simulink model "sysgenTripleBuffer"  (Simulink 7.7)
settings: Solver=ode3  SolverMode=SingleTasking  StartTime=0.0  StopTime=inf  FixedStep=1  RelTol=1e-3
PreLoadFcn:
  | sysgenTripleBuffer_PreloadFcn
undefined symbols (not defined in the file or in its folder): c_hsync, c_image_cols, c_image_rows, c_vsync, c_word_size, gray, pixel_period, videoFrame
libraries: xbsIndex_r4 x101, simulink x4, dspsigattribs x3, dspbuff3 x3, dspmtrx3 x3, xbsCopyrightNotice_r4 x1, vipsnks x1, vipsrcs x1
(part 1 of 2)
settings Model: Creator=arvinds  LastModifiedBy=wayneh
settings OptimizationCC: InlineParams=on
settings ModelReferenceCC: ModelReferenceNumInstancesAllowed=Single
settings SFSimCC: SimParseCustomCode=off

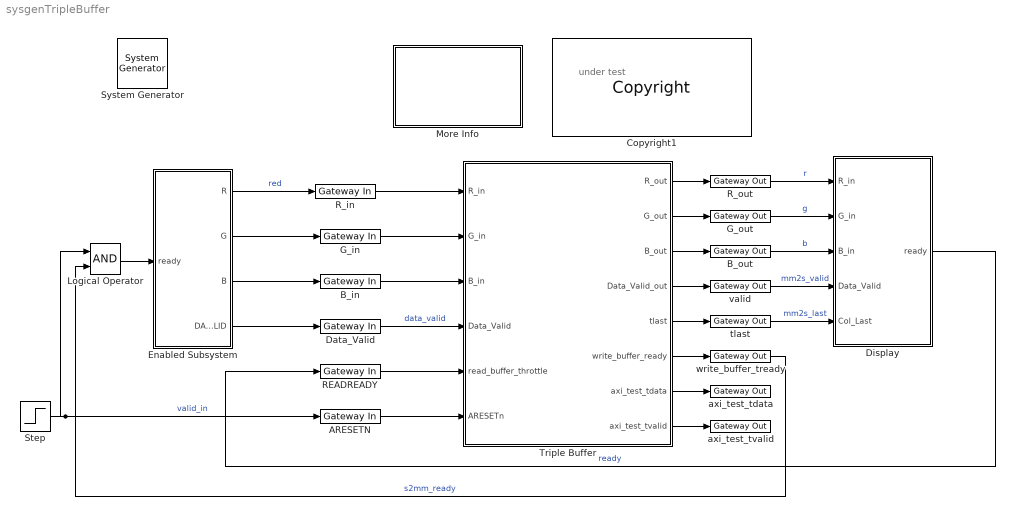
== system sysgenTripleBuffer ==
  note: under test
  " System Generator" : xbsIndex_r4/ System Generator  Tag=genX  SystemSampleTime=-1  xilinxfamily=virtex6  part=xc6vlx240t  speed=-1  package=ff1156  synthesis_tool=XST  clock_wrapper=Clock Enables  directory=./netlist_ml605_v5  proj_type=Project Navigator  Synth_file=XST Defaults  Impl_file=ISE Defaults  testbench=off  simulink_period=1  sysclk_period=20  dcm_input_clock_period=10  incr_netlist=off  trim_vbits=Everywhere in SubSystem  dbl_ovrd=According to Block Masks  core_generation=According to Block Masks  run_coregen=off  deprecated_control=off  eval_field=0  block_type=sysgen
      settings: block_version=12.3
  ARESETN : xbsIndex_r4/Gateway In  gui_display_data_type=Fixed-point  arith_type=Boolean  n_bits=8  bin_pt=0  preci_type=Single  exp_width=8  frac_width=24  quantization="Round  (unbiased: +/- Inf)"  overflow=Saturate  period=pixel_period  dbl_ovrd=off  timing_constraint=None  locs_specified=off  LOCs={}  inherit_from_input=off  UseAsADC=off  ADCChannel='1'  hdl_port=on  block_type=gatewayin
      settings: infoedit="Gateway in block.  Converts inputs of type Simulink integer, double and fixed point to  Xilinx fixed point type.<br><br>Hardware notes:  In hardware these blocks become top level input ports."  block_version=12.3
  B_in : xbsIndex_r4/Gateway In  gui_display_data_type=Fixed-point  arith_type=Unsigned  n_bits=8  bin_pt=0  preci_type=Single  exp_width=8  frac_width=24  quantization="Round  (unbiased: +/- Inf)"  overflow=Saturate  period=pixel_period  dbl_ovrd=off  timing_constraint=None  locs_specified=off  LOCs={}  inherit_from_input=off  UseAsADC=off  ADCChannel='1'  hdl_port=on  block_type=gatewayin
      settings: infoedit="Gateway in block.  Converts inputs of type Simulink integer, double and fixed point to  Xilinx fixed point type.<br><br>Hardware notes:  In hardware these blocks become top level input ports."  block_version=12.3
  B_out : xbsIndex_r4/Gateway Out  inherit_from_input=off  hdl_port=on  timing_constraint=None  locs_specified=off  LOCs={}  UseAsDAC=off  DACChannel='1'  block_type=gatewayout
      settings: infoedit="Gateway out block.  Converts Xilinx fixed point inputs into ouputs of type Simulink integer, double, or fixed point.<br><br>Hardware notes:  In hardware these blocks become top level output ports or are discarded, depending on how they are configured."  block_version=12.3
  Copyright1 : xbsCopyrightNotice_r4/Copyright  copyrighttext="Copyright (c) 2011  by  Xilinx, Inc. All rights reserved.<br><br>This file contains proprietary, confidential information of Xilinx, Inc., is distributed under license from Xilinx, Inc., and may be used, copied and/or disclosed only pursuant to the terms of a valid license agreement with Xilinx, Inc. Xilinx hereby grants you a license to use this file solely for design, simulation, implementation and creation of design files limited to Xilinx devices or technologies. Use with non-Xilinx devices or technologies is expressly prohibited and immediately terminates your license unless covered by a separate agreement.<br><br>Xilinx is providing this design, code, or information \"as-is\" solely for use in developing programs and solutions for Xilinx devices, with no obligation on the part of Xilinx to provide support. By providing this design, code, or information as one possible implementation of this feature, application or standard, Xilinx is making no representation that this implementation is free from any claims of infringement. You are responsible for obtaining any rights you may require for your implementation. Xilinx expressly disclaims any warranty whatsoever with respect to the adequacy of the implementation, including but not limited to any warranties or representations that this implementation is free from claims of infringement, implied warranties of merchantability or fitness for a particular purpose.<br><br>Xilinx products are not intended for use in life support appliances, devices, or systems. Use in such applications is expressly prohibited.<br><br>Any modifications that are made to the Source Code are done at the user's sole risk and will be unsupported.<br><br>This copyright and support notice must be retained as part of this text at all times. (c) Copyright 1995-2011 Xilinx, Inc. All rights reserved."  block_type=copyright
      settings: block_version=10.1.00
  Data_Valid : xbsIndex_r4/Gateway In  gui_display_data_type=Fixed-point  arith_type=Boolean  n_bits=8  bin_pt=0  preci_type=Single  exp_width=8  frac_width=24  quantization="Round  (unbiased: +/- Inf)"  overflow=Saturate  period=pixel_period  dbl_ovrd=off  timing_constraint=None  locs_specified=off  LOCs={}  inherit_from_input=off  UseAsADC=off  ADCChannel='1'  hdl_port=on  block_type=gatewayin
      settings: infoedit="Gateway in block.  Converts inputs of type Simulink integer, double and fixed point to  Xilinx fixed point type.<br><br>Hardware notes:  In hardware these blocks become top level input ports."  block_version=12.3
  Display : Subsystem  mask{im_rows=c_image_rows, im_cols=c_image_cols}
      mask prompts: im_rows "Image Rows"; im_cols "Image Cols"
  Enabled Subsystem : Subsystem  mask{image_cols=c_image_cols, image_rows=c_image_rows, vsync=c_vsync, hsync=c_hsync, videoFrame=videoFrame}
      mask prompts: image_cols "Image Cols"; image_rows "Image Rows"; vsync "VSYNC Size(rows)"; hsync "HSync Size (cols)"; videoFrame "Video Source"
  G_in : xbsIndex_r4/Gateway In  gui_display_data_type=Fixed-point  arith_type=Unsigned  n_bits=8  bin_pt=0  preci_type=Single  exp_width=8  frac_width=24  quantization="Round  (unbiased: +/- Inf)"  overflow=Saturate  period=pixel_period  dbl_ovrd=off  timing_constraint=None  locs_specified=off  LOCs={}  inherit_from_input=off  UseAsADC=off  ADCChannel='1'  hdl_port=on  block_type=gatewayin
      settings: infoedit="Gateway in block.  Converts inputs of type Simulink integer, double and fixed point to  Xilinx fixed point type.<br><br>Hardware notes:  In hardware these blocks become top level input ports."  block_version=12.3
  G_out : xbsIndex_r4/Gateway Out  inherit_from_input=off  hdl_port=on  timing_constraint=None  locs_specified=off  LOCs={}  UseAsDAC=off  DACChannel='1'  block_type=gatewayout
      settings: infoedit="Gateway out block.  Converts Xilinx fixed point inputs into ouputs of type Simulink integer, double, or fixed point.<br><br>Hardware notes:  In hardware these blocks become top level output ports or are discarded, depending on how they are configured."  block_version=12.3
  Logical Operator : Logic  AllPortsSameDT=off  OutDataTypeStr=boolean
  More Info : Subsystem
      mask Display: disp('Double click\n for\n more information.')
  READREADY : xbsIndex_r4/Gateway In  gui_display_data_type=Fixed-point  arith_type=Boolean  n_bits=8  bin_pt=0  preci_type=Single  exp_width=8  frac_width=24  quantization="Round  (unbiased: +/- Inf)"  overflow=Saturate  period=pixel_period  dbl_ovrd=off  timing_constraint=None  locs_specified=off  LOCs={}  inherit_from_input=off  UseAsADC=off  ADCChannel='1'  hdl_port=on  block_type=gatewayin
      settings: infoedit="Gateway in block.  Converts inputs of type Simulink integer, double and fixed point to  Xilinx fixed point type.<br><br>Hardware notes:  In hardware these blocks become top level input ports."  block_version=12.3
  R_in : xbsIndex_r4/Gateway In  gui_display_data_type=Fixed-point  arith_type=Unsigned  n_bits=8  bin_pt=0  preci_type=Single  exp_width=8  frac_width=24  quantization="Round  (unbiased: +/- Inf)"  overflow=Saturate  period=pixel_period  dbl_ovrd=off  timing_constraint=None  locs_specified=off  LOCs={}  inherit_from_input=off  UseAsADC=off  ADCChannel='1'  hdl_port=on  block_type=gatewayin
      settings: infoedit="Gateway in block.  Converts inputs of type Simulink integer, double and fixed point to  Xilinx fixed point type.<br><br>Hardware notes:  In hardware these blocks become top level input ports."  block_version=12.3
  R_out : xbsIndex_r4/Gateway Out  inherit_from_input=off  hdl_port=on  timing_constraint=None  locs_specified=off  LOCs={}  UseAsDAC=off  DACChannel='1'  block_type=gatewayout
      settings: infoedit="Gateway out block.  Converts Xilinx fixed point inputs into ouputs of type Simulink integer, double, or fixed point.<br><br>Hardware notes:  In hardware these blocks become top level output ports or are discarded, depending on how they are configured."  block_version=12.3
  Step : Step  Time=pixel_period*32  SampleTime=pixel_period
  Triple Buffer : Subsystem  mask{c_image_rows=c_image_rows, c_image_cols=c_image_cols, c_word_size=c_word_size}
      mask prompts: c_image_rows "Number of Rows"; c_image_cols "Number of Cols"; c_word_size "Pixel Size(In Bytes)"
  axi_test_tdata : xbsIndex_r4/Gateway Out  inherit_from_input=off  hdl_port=on  timing_constraint=None  locs_specified=off  LOCs={}  UseAsDAC=off  DACChannel='1'  block_type=gatewayout
      settings: infoedit="Gateway out block.  Converts Xilinx fixed point inputs into ouputs of type Simulink integer, double, or fixed point.<br><br>Hardware notes:  In hardware these blocks become top level output ports or are discarded, depending on how they are configured."  block_version=12.3
  axi_test_tvalid : xbsIndex_r4/Gateway Out  inherit_from_input=off  hdl_port=on  timing_constraint=None  locs_specified=off  LOCs={}  UseAsDAC=off  DACChannel='1'  block_type=gatewayout
      settings: infoedit="Gateway out block.  Converts Xilinx fixed point inputs into ouputs of type Simulink integer, double, or fixed point.<br><br>Hardware notes:  In hardware these blocks become top level output ports or are discarded, depending on how they are configured."  block_version=12.3
  tlast : xbsIndex_r4/Gateway Out  inherit_from_input=off  hdl_port=on  timing_constraint=None  locs_specified=off  LOCs={}  UseAsDAC=off  DACChannel='1'  block_type=gatewayout
      settings: infoedit="Gateway out block.  Converts Xilinx fixed point inputs into ouputs of type Simulink integer, double, or fixed point.<br><br>Hardware notes:  In hardware these blocks become top level output ports or are discarded, depending on how they are configured."  block_version=12.3
  valid : xbsIndex_r4/Gateway Out  inherit_from_input=off  hdl_port=on  timing_constraint=None  locs_specified=off  LOCs={}  UseAsDAC=off  DACChannel='1'  block_type=gatewayout
      settings: infoedit="Gateway out block.  Converts Xilinx fixed point inputs into ouputs of type Simulink integer, double, or fixed point.<br><br>Hardware notes:  In hardware these blocks become top level output ports or are discarded, depending on how they are configured."  block_version=12.3
  write_buffer_tready : xbsIndex_r4/Gateway Out  inherit_from_input=off  hdl_port=on  timing_constraint=None  locs_specified=off  LOCs={}  UseAsDAC=off  DACChannel='1'  block_type=gatewayout
      settings: infoedit="Gateway out block.  Converts Xilinx fixed point inputs into ouputs of type Simulink integer, double, or fixed point.<br><br>Hardware notes:  In hardware these blocks become top level output ports or are discarded, depending on how they are configured."  block_version=12.3
  wires:
  Step/1 -> Logical Operator/1, ARESETN/1  "valid_in"
  Enabled Subsystem/1(R) -> R_in/1  "red"
  Enabled Subsystem/2(G) -> G_in/1
  Enabled Subsystem/3(B) -> B_in/1
  R_out/1 -> Display/1(R_in)  "r"
  G_out/1 -> Display/2(G_in)  "g"
  B_out/1 -> Display/3(B_in)  "b"
  valid/1 -> Display/4(Data_Valid)  "mm2s_valid"
  tlast/1 -> Display/5(Col_Last)  "mm2s_last"
  write_buffer_tready/1 -> Logical Operator/2  "s2mm_ready"
  Enabled Subsystem/4(DATA_VALID) -> Data_Valid/1
  Logical Operator/1 -> Enabled Subsystem/1(ready)
  Display/1(ready) -> READREADY/1  "ready"
  R_in/1 -> Triple Buffer/1(R_in)
  G_in/1 -> Triple Buffer/2(G_in)
  B_in/1 -> Triple Buffer/3(B_in)
  Data_Valid/1 -> Triple Buffer/4(Data_Valid)  "data_valid"
  Triple Buffer/3(B_out) -> B_out/1
  Triple Buffer/4(Data_Valid_out) -> valid/1
  Triple Buffer/5(tlast) -> tlast/1
  Triple Buffer/6(write_buffer_ready) -> write_buffer_tready/1
  ARESETN/1 -> Triple Buffer/6(ARESETn)
  Triple Buffer/1(R_out) -> R_out/1
  Triple Buffer/2(G_out) -> G_out/1
  READREADY/1 -> Triple Buffer/5(read_buffer_throttle)
  Triple Buffer/7(axi_test_tdata) -> axi_test_tdata/1
  Triple Buffer/8(axi_test_tvalid) -> axi_test_tvalid/1

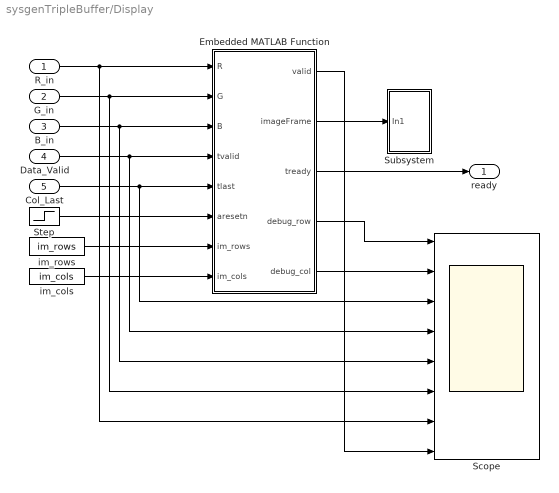
== system sysgenTripleBuffer/Display ==
  R_in : Inport
  G_in : Inport  Port=2
  B_in : Inport  Port=3
  Data_Valid : Inport  Port=4
  Col_Last : Inport  Port=5
  Embedded MATLAB Function : Stateflow chart  TreatAsAtomicUnit=on
  Scope : Scope  NumInputPorts=8
      settings: YMin=7.6~17.5~-1~0.95~-1~-1~-1~-1  YMax=8.4~35~1~1.05~1~1~1~1
  Step : Step  Time=pixel_period  SampleTime=pixel_period
  Subsystem : Subsystem
  im_cols : Constant  Value=im_cols
  im_rows : Constant  Value=im_rows
  ready : Outport
  wires:
  Step/1 -> Embedded MATLAB Function/6(aresetn)
  Embedded MATLAB Function/1(valid) -> Scope/8
  Embedded MATLAB Function/2(imageFrame) -> Subsystem/1(In1)
  R_in/1 -> Embedded MATLAB Function/1(R), Scope/7
  G_in/1 -> Embedded MATLAB Function/2(G), Scope/6
  B_in/1 -> Embedded MATLAB Function/3(B), Scope/5
  Col_Last/1 -> Embedded MATLAB Function/5(tlast), Scope/3
  Data_Valid/1 -> Embedded MATLAB Function/4(tvalid), Scope/4
  Embedded MATLAB Function/3(tready) -> ready/1
  im_rows/1 -> Embedded MATLAB Function/7(im_rows)
  im_cols/1 -> Embedded MATLAB Function/8(im_cols)
  Embedded MATLAB Function/4(debug_row) -> Scope/1
  Embedded MATLAB Function/5(debug_col) -> Scope/2

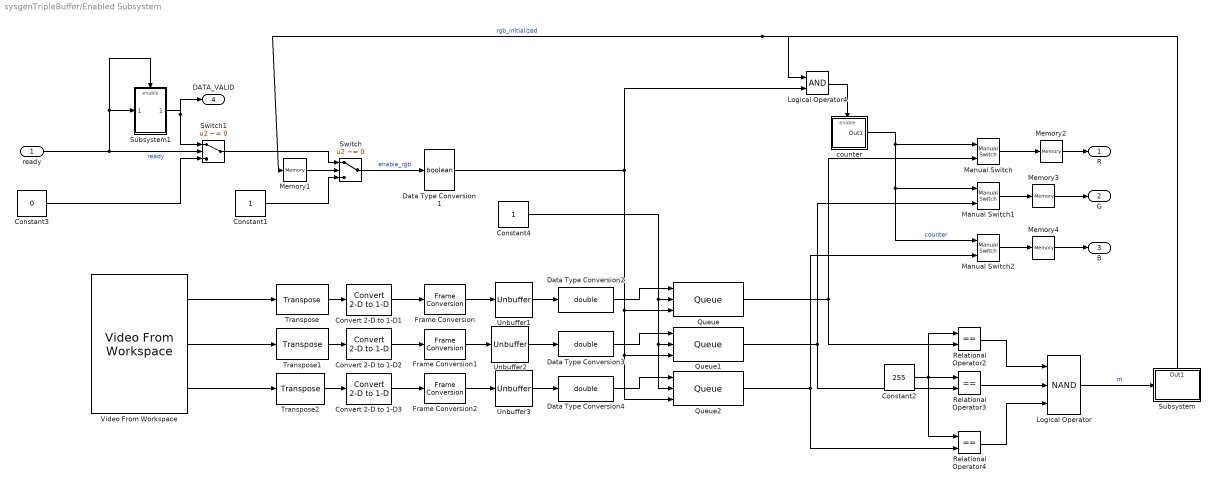
== system sysgenTripleBuffer/Enabled Subsystem ==
  ready : Inport
  Constant1 : Constant
  Constant2 : Constant  Value=255
  Constant3 : Constant  Value=0
  Constant4 : Constant  OutDataTypeStr=boolean
  Convert 2-D to 1-D1 : dspsigattribs/Convert 2-D to 1-D  SystemSampleTime=-1
  Convert 2-D to 1-D2 : dspsigattribs/Convert 2-D to 1-D  SystemSampleTime=-1
  Convert 2-D to 1-D3 : dspsigattribs/Convert 2-D to 1-D  SystemSampleTime=-1
  Data Type Conversion1 : DataTypeConversion  OutDataTypeStr=boolean
  Data Type Conversion2 : DataTypeConversion  OutDataTypeStr=double
  Data Type Conversion3 : DataTypeConversion  OutDataTypeStr=double
  Data Type Conversion4 : DataTypeConversion  OutDataTypeStr=double
  Frame Conversion : FrameConversion
  Frame Conversion1 : FrameConversion
  Frame Conversion2 : FrameConversion
  Logical Operator : Logic  Operator=NAND  Inputs=3  AllPortsSameDT=off  OutDataTypeStr=boolean
  Logical Operator4 : Logic  AllPortsSameDT=off  OutDataTypeStr=boolean
  Manual Switch : simulink/Signal Routing/Manual Switch  SystemSampleTime=-1  sw=0  action=0  varsize=off
  Manual Switch1 : simulink/Signal Routing/Manual Switch  SystemSampleTime=-1  sw=0  action=0  varsize=off
  Manual Switch2 : simulink/Signal Routing/Manual Switch  SystemSampleTime=-1  sw=0  action=0  varsize=off
  Memory{1..4} (4 alike) : Memory  InheritSampleTime=on  LinearizeMemory=on  LinearizeAsDelay=on
  Queue : dspbuff3/Queue  depth=image_cols*image_rows*10  trigger=Non-zero sample  overflow=Dynamic reallocation  pes=Warning  eso=off  fso=off  nso=off  clr=off  clrOutport=off  adf=on
  Queue1 : dspbuff3/Queue  depth=image_cols*image_rows*10  trigger=Non-zero sample  overflow=Dynamic reallocation  pes=Warning  eso=off  fso=off  nso=off  clr=off  clrOutport=off  adf=on
  Queue2 : dspbuff3/Queue  depth=image_cols*image_rows*10  trigger=Non-zero sample  overflow=Dynamic reallocation  pes=Warning  eso=off  fso=off  nso=off  clr=off  clrOutport=off  adf=on
  Relational Operator2 : RelationalOperator  Operator===  OutDataTypeStr=boolean
  Relational Operator3 : RelationalOperator  Operator===  OutDataTypeStr=boolean
  Relational Operator4 : RelationalOperator  Operator===  OutDataTypeStr=boolean
  Subsystem : Subsystem
  Subsystem1 : Subsystem
  Switch : Switch  Criteria=u2 ~= 0
  Switch1 : Switch  Criteria=u2 ~= 0
  Transpose : dspmtrx3/Transpose  SystemSampleTime=-1  Hermitian=off  overflowFlag=off
  Transpose1 : dspmtrx3/Transpose  SystemSampleTime=-1  Hermitian=off  overflowFlag=off
  Transpose2 : dspmtrx3/Transpose  SystemSampleTime=-1  Hermitian=off  overflowFlag=off
  Unbuffer1 : Unbuffer
  Unbuffer2 : Unbuffer
  Unbuffer3 : Unbuffer
  Video From Workspace : vipsrcs/Video From Workspace  signal=videoFrame  Ts=image_cols*image_rows  finalout=Obsolete  finaloutActive=Cyclic repetition  imagePorts=Separate color signals  OutPortLabels=R|G|B
  counter : Subsystem
  R : Outport
  G : Outport  Port=2
  B : Outport  Port=3
  DATA_VALID : Outport  Port=4  SampleTime=pixel_period
  wires:
  Relational Operator2/1 -> Logical Operator/1
  Relational Operator3/1 -> Logical Operator/2
  Relational Operator4/1 -> Logical Operator/3
  Subsystem/1(Out1) -> Logical Operator4/1, Memory1/1  "rgb_initialized"
  Constant1/1 -> Switch/3
  Switch/1 -> Data Type Conversion1/1  "enable_rgb"
  Manual Switch/1 -> Memory2/1
  Manual Switch1/1 -> Memory3/1
  Manual Switch2/1 -> Memory4/1
  counter/1(Out1) -> Manual Switch/1, Manual Switch1/1, Manual Switch2/1  "counter"
  Logical Operator4/1 -> counter/Enable
  Logical Operator/1 -> Subsystem/Enable  "m"
  Constant2/1 -> Relational Operator3/1, Relational Operator2/1, Relational Operator4/1
  Memory1/1 -> Switch/2
  ready/1 -> Subsystem1/1(In1), Subsystem1/Enable, Switch1/2  "ready"
  Subsystem1/1(Out1) -> Switch1/1, DATA_VALID/1
  Constant3/1 -> Switch1/3
  Switch1/1 -> Switch/1
  Convert 2-D to 1-D3/1 -> Frame Conversion2/1
  Transpose2/1 -> Convert 2-D to 1-D3/1
  Convert 2-D to 1-D2/1 -> Frame Conversion1/1
  Transpose1/1 -> Convert 2-D to 1-D2/1
  Convert 2-D to 1-D1/1 -> Frame Conversion/1
  Transpose/1 -> Convert 2-D to 1-D1/1
  Video From Workspace/1 -> Transpose/1
  Video From Workspace/2 -> Transpose1/1
  Video From Workspace/3 -> Transpose2/1
  Data Type Conversion1/1 -> Logical Operator4/2, Queue/3, Queue1/3, Queue2/3
  Data Type Conversion2/1 -> Queue/1
  Data Type Conversion3/1 -> Queue1/1
  Data Type Conversion4/1 -> Queue2/1
  Queue/1 -> Relational Operator2/2, Manual Switch/2
  Queue1/1 -> Relational Operator3/2, Manual Switch1/2
  Queue2/1 -> Relational Operator4/2, Manual Switch2/2
  Constant4/1 -> Queue/2, Queue1/2, Queue2/2
  Frame Conversion/1 -> Unbuffer1/1
  Frame Conversion1/1 -> Unbuffer2/1
  Frame Conversion2/1 -> Unbuffer3/1
  Unbuffer1/1 -> Data Type Conversion2/1
  Unbuffer2/1 -> Data Type Conversion3/1
  Unbuffer3/1 -> Data Type Conversion4/1
  Memory2/1 -> R/1
  Memory3/1 -> G/1
  Memory4/1 -> B/1

== system sysgenTripleBuffer/More Info ==
  note: Triple Buffer Demo
  note: This model implements a triple buffer controller that controls how frames are written to an external memory and read using a VDMA Interface 4.0 .
      | As the name suggests, triple buffer is a methodology used to synchronize data transfer between a writing device and reading device using
      | three buffers. The writing device does not write to the buffer that is being used by the reading device. Instead the writing device writes alternatively
      | to two buffers available to it. When the reading device has finished reading the buffer is swapped with the buffer that was last written to and the
      | process is continued. This methodology is generally used in graphics processing where the graphics processor is the writing device and
      | the display device is the reading device.
      |
      | The design can be netlisted using HDL Netlist in which case the VDMA Interface 4.0  block will be translated into top level gateways. Furthermore,
      | xlVDMACreateProject function can be used to create an ISE project to stitch SysGen design with VDMA Interface 3.0  & External Memory in XPS.
      | For more information please type the following in matlab console :
      | >>help xlVDMACreateProject
      |
      | Please refer to in case stateflow block compiler setup error.
      | http://www.mathworks.com/help/toolbox/stateflow/gs/bqnop_7-1.html

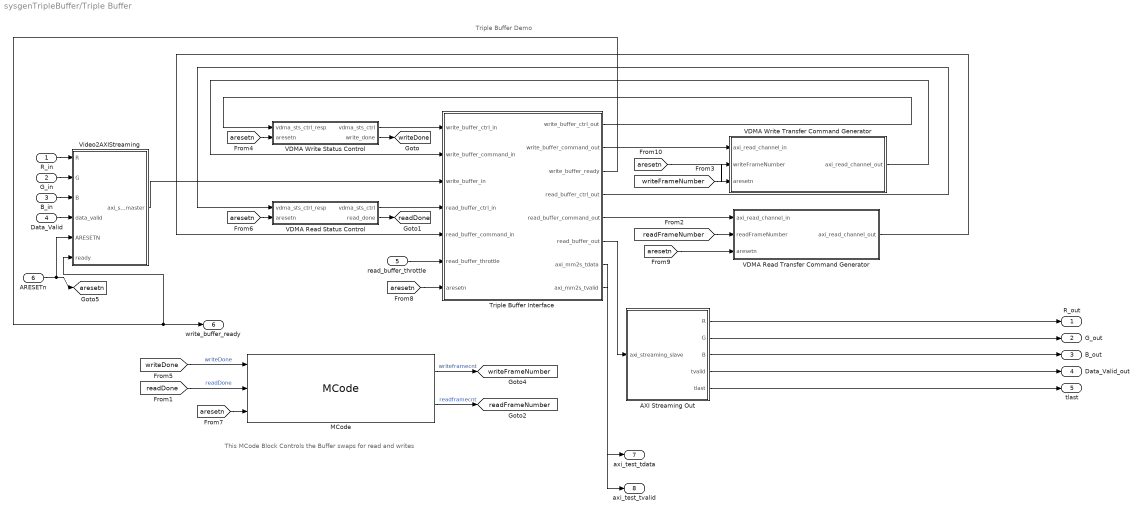
== system sysgenTripleBuffer/Triple Buffer ==
  note: This MCode Block Controls the Buffer swaps
      | for read and writes
  note: Triple Buffer Demo
  R_in : Inport
  G_in : Inport  Port=2
  B_in : Inport  Port=3
  Data_Valid : Inport  Port=4
  read_buffer_throttle : Inport  Port=5
  ARESETn : Inport  Port=6
  AXI Streaming Out : Subsystem
  MCode : xbsIndex_r4/MCode  mfname=xlTripleBufferAddressController  explicit_period=on  period=pixel_period  inputsTable={'boundInpExpr'=>['','',''],'inputs'=>['writeDone','readDone','aresetn']}  outputsTable={'outputs'=>['writeFrameNumber','readFrameNumber'],'suppressOut'=>['off','off']}  dbl_ovrd=off  enable_stdout=off  enable_debug=off  suppress_output=on  defparams={}  hide_port_list={}  block_type=mcode
      settings: block_version=12.3
  Triple Buffer Interface : Subsystem
  VDMA Read Status Control : Subsystem
  VDMA Read Transfer Command Generator : Subsystem
  VDMA Write Status Control : Subsystem
  VDMA Write Transfer Command Generator : Subsystem
  Video2AXIStreaming : Subsystem
  R_out : Outport
  G_out : Outport  Port=2
  B_out : Outport  Port=3
  Data_Valid_out : Outport  Port=4
  tlast : Outport  Port=5
  write_buffer_ready : Outport  Port=6
  axi_test_tdata : Outport  Port=7
  axi_test_tvalid : Outport  Port=8
  tag scope: aresetn=global, readDone=global, readFrameNumber=global, writeDone=global, writeFrameNumber=global
  wires:
  VDMA Write Status Control/1(vdma_sts_ctrl) -> Triple Buffer Interface/1(write_buffer_ctrl_in)
  Triple Buffer Interface/1(write_buffer_ctrl_out) -> VDMA Write Status Control/1(vdma_sts_ctrl_resp)
  VDMA Read Status Control/1(vdma_sts_ctrl) -> Triple Buffer Interface/4(read_buffer_ctrl_in)
  Triple Buffer Interface/4(read_buffer_ctrl_out) -> VDMA Read Status Control/1(vdma_sts_ctrl_resp)
  VDMA Write Status Control/2(write_done) -> [writeDone]
  VDMA Read Status Control/2(read_done) -> [readDone]
  [writeDone] -> MCode/1  "writeDone"
  [readDone] -> MCode/2  "readDone"
  Triple Buffer Interface/2(write_buffer_command_out) -> VDMA Write Transfer Command Generator/1(axi_read_channel_in)
  VDMA Write Transfer Command Generator/1(axi_read_channel_out) -> Triple Buffer Interface/2(write_buffer_command_in)
  Triple Buffer Interface/5(read_buffer_command_out) -> VDMA Read Transfer Command Generator/1(axi_read_channel_in)
  [readFrameNumber] -> VDMA Read Transfer Command Generator/2(readFrameNumber)
  [writeFrameNumber] -> VDMA Write Transfer Command Generator/2(writeFrameNumber)
  MCode/1 -> [writeFrameNumber]  "writeframecnt"
  [aresetn] -> VDMA Write Status Control/2(aresetn)
  ARESETn/1 -> Video2AXIStreaming/5(ARESETN), [aresetn]
  VDMA Read Transfer Command Generator/1(axi_read_channel_out) -> Triple Buffer Interface/5(read_buffer_command_in)
  [aresetn] -> MCode/3
  [aresetn] -> Triple Buffer Interface/7(aresetn)
  [aresetn] -> VDMA Write Transfer Command Generator/3(aresetn)
  [aresetn] -> VDMA Read Transfer Command Generator/3(aresetn)
  MCode/2 -> [readFrameNumber]  "readframecnt"
  [aresetn] -> VDMA Read Status Control/2(aresetn)
  Video2AXIStreaming/1(axi_streaming_master) -> Triple Buffer Interface/3(write_buffer_in)
  Triple Buffer Interface/6(read_buffer_out) -> AXI Streaming Out/1(axi_streaming_slave)
  AXI Streaming Out/1(R) -> R_out/1
  AXI Streaming Out/2(G) -> G_out/1
  AXI Streaming Out/3(B) -> B_out/1
  AXI Streaming Out/5(tlast) -> tlast/1
  AXI Streaming Out/4(tvalid) -> Data_Valid_out/1
  R_in/1 -> Video2AXIStreaming/1(R)
  G_in/1 -> Video2AXIStreaming/2(G)
  B_in/1 -> Video2AXIStreaming/3(B)
  Data_Valid/1 -> Video2AXIStreaming/4(data_valid)
  read_buffer_throttle/1 -> Triple Buffer Interface/6(read_buffer_throttle)
  Triple Buffer Interface/3(write_buffer_ready) -> write_buffer_ready/1, Video2AXIStreaming/6(ready)
  Triple Buffer Interface/7(axi_mm2s_tdata) -> axi_test_tdata/1
  Triple Buffer Interface/8(axi_mm2s_tvalid) -> axi_test_tvalid/1

== system sysgenTripleBuffer/Display/Subsystem ==
  In1 : Inport
  Video Viewer_simulation : vipsnks/Video Viewer  inputType=Obsolete7b  imagePorts=One multidimensional signal  useColorMap=off  colormapValue=gray(256)  specRange=off  minInputVal=0  maxInputVal=255  FigPos=[590 848 651 583]  AxisZoom=on  trueSizedOnce=off  OpenAtMdlStart=on
  wires:
  In1/1 -> Video Viewer_simulation/1

== system sysgenTripleBuffer/Enabled Subsystem/Subsystem ==
  Enable : EnablePort
  Step : Step  Time=0  SampleTime=pixel_period
  Out1 : Outport
  wires:
  Step/1 -> Out1/1

== system sysgenTripleBuffer/Enabled Subsystem/Subsystem1 ==
  In1 : Inport
  Enable : EnablePort
  Memory2 : Memory  InheritSampleTime=on  LinearizeAsDelay=on
  Out1 : Outport
  wires:
  In1/1 -> Memory2/1
  Memory2/1 -> Out1/1

== system sysgenTripleBuffer/Enabled Subsystem/counter ==
  Enable : EnablePort
  Counter Limited : simulink/Sources/Counter Limited  SystemSampleTime=-1  uplimit=159  tsamp=-1
  Out1 : Outport  InitialOutput=0
  wires:
  Counter Limited/1 -> Out1/1

== system sysgenTripleBuffer/Triple Buffer/AXI Streaming Out ==
  axi_streaming_slave : Inport
  BitBasher : xbsIndex_r4/BitBasher  bitexpr=|  display_expr=off  sr_1=1  arith_type1=Unsigned  bin_pt1=0  sr_2=2  arith_type2=Unsigned  bin_pt2=0  sr_3=3  arith_type3=Unsigned  bin_pt3=0  sr_4=4  arith_type4=Unsigned  bin_pt4=0  dbl_ovrd=off  block_type=bitbasher
      | <!DOCTYPE HTML PUBLIC "-//W3C//DTD HTML 4.0//EN" "http://www.w3.org/TR/REC-html40/strict.dtd">
      | <html><head><meta name="qrichtext" content="1" /><style type="text/css">
      | p, li { white-space: pre-wrap; }
      | </style></head><body style=" font-family:'MS Shell Dlg 2'; font-size:8.25pt; font-weight:400; font-style:normal;">
      | <p style=" margin-top:12px; margin-bottom:12px; margin-left:0px; margin-right:0px; -qt-block-indent:0; text-indent:0px; font-family:'MS Shell Dlg'; font-size:8pt;">R={tdata[23:16]}<br />G={tdata[15:8]}<br />B={tdata[7:0]}</p></body></html>
      settings: block_version=13.3
  Bus Selector6 : BusSelector  OutputSignals=signal1,signal2,signal3,signal4
  Terminator1 : Terminator
  R : Outport
  G : Outport  Port=2
  B : Outport  Port=3
  tvalid : Outport  Port=4
  tlast : Outport  Port=5
  wires:
  axi_streaming_slave/1 -> Bus Selector6/1
  Bus Selector6/3 -> tvalid/1  "<signal3>"
  Bus Selector6/4 -> tlast/1  "<signal4>"
  Bus Selector6/2 -> Terminator1/1  "<signal2>"
  Bus Selector6/1 -> BitBasher/1  "<signal1>"
  BitBasher/1 -> R/1
  BitBasher/2 -> G/1
  BitBasher/3 -> B/1

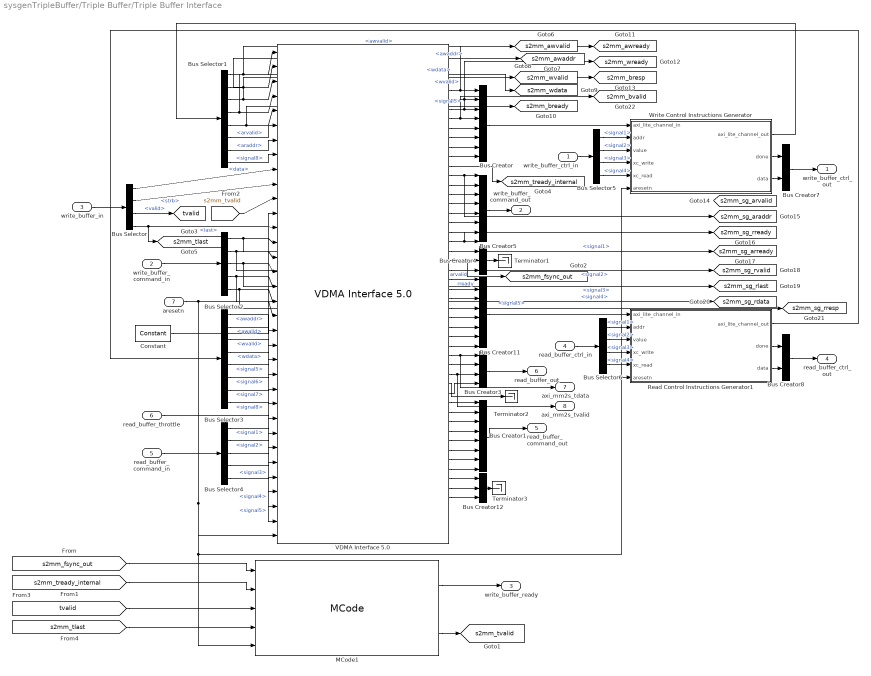
== system sysgenTripleBuffer/Triple Buffer/Triple Buffer Interface ==
  write_buffer_ctrl_in : Inport
  write_buffer_command_in : Inport  Port=2
  write_buffer_in : Inport  Port=3
  read_buffer_ctrl_in : Inport  Port=4
  read_buffer_command_in : Inport  Port=5
  read_buffer_throttle : Inport  Port=6
  aresetn : Inport  Port=7
  Bus Creator{,1,5,11} (4 alike) : BusCreator  Inputs=8
  Bus Creator12 : BusCreator  Inputs=3
  Bus Creator3 : BusCreator
  Bus Creator4 : BusCreator  Inputs=3
  Bus Creator7 : BusCreator  Inputs=2
  Bus Creator8 : BusCreator  Inputs=2
  Bus Selector : BusSelector  OutputSignals=data,strb,valid,last
  Bus Selector1 : BusSelector  OutputSignals=awvalid,awaddr,wvalid,wdata,signal5,arvalid,araddr,signal8
  Bus Selector2 : BusSelector  OutputSignals=signal1,signal2,signal3,signal4,signal5
  Bus Selector3 : BusSelector  OutputSignals=awaddr,awalid,wvalid,wdata,signal5,signal6,signal7,signal8
  Bus Selector4 : BusSelector  OutputSignals=signal1,signal2,signal3,signal4,signal5
  Bus Selector5 : BusSelector  OutputSignals=signal1,signal2,signal3,signal4
  Bus Selector6 : BusSelector  OutputSignals=signal1,signal2,signal3,signal4
  Constant : xbsIndex_r4/Constant  const=1  gui_display_data_type=Fixed-point  arith_type=Unsigned  n_bits=1  bin_pt=0  preci_type=Single  exp_width=8  frac_width=24  explicit_period=on  period=1  equ=P=C  opselect=C  inp2=PCIN>>17  opr=+  inp1=P  carry=CIN  dbl_ovrd=off  block_type=constant
      settings: block_version=13.4
  MCode1 : xbsIndex_r4/MCode  mfname=xlTreadyWorkaroundS2MM  explicit_period=off  period=pixel_period  inputsTable={'boundInpExpr'=>['','','','','','c_image_rows'],'inputs'=>['s2mm_fsync_out','s2mm_tready','tvalid','s2mm_tlast','aresetn','VSIZE']}  outputsTable={'outputs'=>['tready','s2mm_tvalid'],'suppressOut'=>['off','off']}  dbl_ovrd=off  enable_stdout=off  enable_debug=off  suppress_output=on  defparams={'VSIZE',c_image_rows}  hide_port_list={}  block_type=mcode
      settings: block_version=12.3
  Read Control Instructions Generator1 : Subsystem
  Terminator1 : Terminator
  Terminator2 : Terminator
  Terminator3 : Terminator
  "VDMA Interface 5.0 " : xbsIndex_r4/VDMA Interface 5.0   c_mem_size=64MB  c_number_of_vdma_if=2  c_stream_if_configuration_1=Slave  c_no_of_frames_1=c_num_fstores  c_use_fsync_1=off  c_flush_on_fsync_1=off  c_use_sg_engine_1=on  c_video_prm_read_1=on  c_m_axis_mm2s_data_width_1=32  c_m_axis_mm2s_frame_sync_tuser_1=off  c_mm2s_linebuffer_depth_1=0  c_mm2s_linebuffer_threshold_1=1  c_s_axis_s2mm_data_width_1=32  c_s_axis_s2mm_frame_sync_tuser_1=off  c_s2mm_linebuffer_depth_1=0  c_s2mm_linebuffer_threshold_1=1  c_stream_if_configuration_2=Master  c_no_of_frames_2=c_num_fstores  c_use_fsync_2=off  c_flush_on_fsync_2=off  c_use_sg_engine_2=on  c_video_prm_read_2=on  c_m_axis_mm2s_data_width_2=32  c_m_axis_mm2s_frame_sync_tuser_2=off  c_mm2s_linebuffer_depth_2=0  c_mm2s_linebuffer_threshold_2=1  c_s_axis_s2mm_data_width_2=32  c_s_axis_s2mm_frame_sync_tuser_2=off  c_s2mm_linebuffer_depth_2=0  c_s2mm_linebuffer_threshold_2=1  c_stream_if_configuration_3=Master/Slave  c_no_of_frames_3=3  c_use_fsync_3=off  c_flush_on_fsync_3=off  c_use_sg_engine_3=off  c_video_prm_read_3=on  c_m_axis_mm2s_data_width_3=32  c_m_axis_mm2s_frame_sync_tuser_3=off  c_mm2s_linebuffer_depth_3=0  c_mm2s_linebuffer_threshold_3=1  c_s_axis_s2mm_data_width_3=32  c_s_axis_s2mm_frame_sync_tuser_3=off  c_s2mm_linebuffer_depth_3=0  c_s2mm_linebuffer_threshold_3=1  c_stream_if_configuration_4=Master/Slave  c_no_of_frames_4=3  c_use_fsync_4=off  c_flush_on_fsync_4=off  c_use_sg_engine_4=off  c_video_prm_read_4=on  c_m_axis_mm2s_data_width_4=32  c_m_axis_mm2s_frame_sync_tuser_4=off  c_mm2s_linebuffer_depth_4=0  c_mm2s_linebuffer_threshold_4=1  c_s_axis_s2mm_data_width_4=32  c_s_axis_s2mm_frame_sync_tuser_4=off  c_s2mm_linebuffer_depth_4=0  c_s2mm_linebuffer_threshold_4=1  simulation_model='emi_v5_0:EMI_v5_0_Model'  block_type=vdma
      settings: infoedit="This is a bit-accurate simulation model for multiple AXI VDMA external memory interfaces.  Netlisting will generate the port interface that can be attached to the VDMA IP.  This block is currently in beta."  block_version=13.4
  Write Control Instructions Generator : Subsystem
  write_buffer_ctrl_out : Outport
  write_buffer_command_out : Outport  Port=2
  write_buffer_ready : Outport  Port=3
  read_buffer_ctrl_out : Outport  Port=4
  read_buffer_command_out : Outport  Port=5
  read_buffer_out : Outport  Port=6
  axi_mm2s_tdata : Outport  Port=7
  axi_mm2s_tvalid : Outport  Port=8
  tag scope: s2mm_awaddr=global, s2mm_awready=global, s2mm_awvalid=global, s2mm_bready=global, s2mm_bresp=global, s2mm_bvalid=global, s2mm_fsync_out=global, s2mm_sg_araddr=global, s2mm_sg_arready=global, s2mm_sg_arvalid=global, s2mm_sg_rdata=global, s2mm_sg_rlast=global, s2mm_sg_rready=global, s2mm_sg_rresp=global, s2mm_sg_rvalid=global, s2mm_tlast=global, s2mm_tready_internal=global, s2mm_tvalid=global, s2mm_wdata=global, s2mm_wready=global, s2mm_wvalid=global, tvalid=global
  wires:
  Bus Selector/1 -> "VDMA Interface 5.0 "/9  "<data>"
  Bus Selector/2 -> "VDMA Interface 5.0 "/10  "<strb>"
  Bus Selector/4 -> [s2mm_tlast], "VDMA Interface 5.0 "/13  "<last>"
  write_buffer_command_in/1 -> Bus Selector2/1
  Bus Creator/1 -> Write Control Instructions Generator/1(axi_lite_channel_in)
  Bus Creator5/1 -> write_buffer_command_out/1
  write_buffer_in/1 -> Bus Selector/1
  Write Control Instructions Generator/1(axi_lite_channel_out) -> Bus Selector1/1
  Bus Selector5/1 -> Write Control Instructions Generator/2(addr)  "<signal1>"
  Bus Selector5/4 -> Write Control Instructions Generator/5(xc_read)  "<signal4>"
  Bus Selector5/2 -> Write Control Instructions Generator/3(value)  "<signal2>"
  Bus Selector5/3 -> Write Control Instructions Generator/4(xc_write)  "<signal3>"
  write_buffer_ctrl_in/1 -> Bus Selector5/1
  Bus Creator11/1 -> Read Control Instructions Generator1/1(axi_lite_channel_in)
  Bus Selector6/1 -> Read Control Instructions Generator1/2(addr)  "<signal1>"
  Bus Selector6/2 -> Read Control Instructions Generator1/3(value)  "<signal2>"
  Bus Selector6/3 -> Read Control Instructions Generator1/4(xc_write)  "<signal3>"
  Bus Selector6/4 -> Read Control Instructions Generator1/5(xc_read)  "<signal4>"
  read_buffer_ctrl_in/1 -> Bus Selector6/1
  Read Control Instructions Generator1/1(axi_lite_channel_out) -> Bus Selector3/1
  read_buffer_command_in/1 -> Bus Selector4/1
  Bus Creator1/1 -> read_buffer_command_out/1
  Bus Creator3/1 -> read_buffer_out/1
  Write Control Instructions Generator/3(data) -> Bus Creator7/2
  Write Control Instructions Generator/2(done) -> Bus Creator7/1
  Bus Creator7/1 -> write_buffer_ctrl_out/1
  Read Control Instructions Generator1/2(done) -> Bus Creator8/1
  Read Control Instructions Generator1/3(data) -> Bus Creator8/2
  Bus Creator8/1 -> read_buffer_ctrl_out/1
  "VDMA Interface 5.0 "/1 -> Bus Creator/1, [s2mm_awready]
  "VDMA Interface 5.0 "/2 -> Bus Creator/2, [s2mm_wready]
  "VDMA Interface 5.0 "/3 -> Bus Creator/3, [s2mm_bresp]
  "VDMA Interface 5.0 "/4 -> Bus Creator/4, [s2mm_bvalid]
  "VDMA Interface 5.0 "/5 -> Bus Creator/5
  "VDMA Interface 5.0 "/6 -> Bus Creator/6
  "VDMA Interface 5.0 "/7 -> Bus Creator/7
  "VDMA Interface 5.0 "/8 -> Bus Creator/8
  Bus Creator12/1 -> Terminator3/1
  "VDMA Interface 5.0 "/11 -> Bus Creator5/2
  "VDMA Interface 5.0 "/12 -> Bus Creator5/3
  "VDMA Interface 5.0 "/13 -> Bus Creator5/4
  "VDMA Interface 5.0 "/14 -> Bus Creator5/5
  "VDMA Interface 5.0 "/15 -> Bus Creator5/6
  "VDMA Interface 5.0 "/16 -> Bus Creator5/7
  "VDMA Interface 5.0 "/17 -> Bus Creator5/8, [s2mm_sg_rready]
  "VDMA Interface 5.0 "/18 -> Bus Creator4/1
  "VDMA Interface 5.0 "/19 -> Bus Creator4/2, [s2mm_fsync_out]
  "VDMA Interface 5.0 "/20 -> Bus Creator4/3  "arvalid"
  "VDMA Interface 5.0 "/21 -> Bus Creator11/1  "rready"
  "VDMA Interface 5.0 "/22 -> Bus Creator11/2
  "VDMA Interface 5.0 "/23 -> Bus Creator11/3
  "VDMA Interface 5.0 "/24 -> Bus Creator11/4
  "VDMA Interface 5.0 "/25 -> Bus Creator11/5
  "VDMA Interface 5.0 "/26 -> Bus Creator11/6
  "VDMA Interface 5.0 "/27 -> Bus Creator11/7
  "VDMA Interface 5.0 "/10 -> Bus Creator5/1, [s2mm_sg_araddr]
  "VDMA Interface 5.0 "/28 -> Bus Creator11/8
  "VDMA Interface 5.0 "/29 -> Bus Creator3/1, axi_mm2s_tdata/1
  "VDMA Interface 5.0 "/30 -> Bus Creator3/2
  "VDMA Interface 5.0 "/31 -> Bus Creator3/3, axi_mm2s_tvalid/1
  "VDMA Interface 5.0 "/33 -> Bus Creator3/4
  "VDMA Interface 5.0 "/34 -> Bus Creator1/1
  "VDMA Interface 5.0 "/35 -> Bus Creator1/2
  "VDMA Interface 5.0 "/36 -> Bus Creator1/3
  "VDMA Interface 5.0 "/37 -> Bus Creator1/4
  "VDMA Interface 5.0 "/38 -> Bus Creator1/5
  "VDMA Interface 5.0 "/39 -> Bus Creator1/6
  "VDMA Interface 5.0 "/40 -> Bus Creator1/7
  "VDMA Interface 5.0 "/41 -> Bus Creator1/8
  "VDMA Interface 5.0 "/42 -> Bus Creator12/1
  "VDMA Interface 5.0 "/43 -> Bus Creator12/2
  "VDMA Interface 5.0 "/44 -> Bus Creator12/3
  Bus Selector1/1 -> [s2mm_awvalid], "VDMA Interface 5.0 "/1  "<awvalid>"
  Bus Selector1/2 -> [s2mm_awaddr], "VDMA Interface 5.0 "/2  "<awaddr>"
  Bus Selector1/3 -> [s2mm_wvalid], "VDMA Interface 5.0 "/3  "<wvalid>"
  Bus Selector1/4 -> [s2mm_wdata], "VDMA Interface 5.0 "/4  "<wdata>"
  Bus Selector1/5 -> [s2mm_bready], "VDMA Interface 5.0 "/5  "<signal5>"
  Bus Selector1/6 -> "VDMA Interface 5.0 "/6  "<arvalid>"
  Bus Selector1/7 -> "VDMA Interface 5.0 "/7  "<araddr>"
  Bus Selector1/8 -> "VDMA Interface 5.0 "/8  "<signal8>"
  Bus Selector2/1 -> [s2mm_sg_arready], "VDMA Interface 5.0 "/14  "<signal1>"
  Bus Selector2/2 -> [s2mm_sg_rvalid], "VDMA Interface 5.0 "/15  "<signal2>"
  Bus Selector2/3 -> [s2mm_sg_rlast], "VDMA Interface 5.0 "/16  "<signal3>"
  Bus Selector2/4 -> [s2mm_sg_rdata], "VDMA Interface 5.0 "/17  "<signal4>"
  Bus Selector2/5 -> [s2mm_sg_rresp], "VDMA Interface 5.0 "/18  "<signal5>"
  aresetn/1 -> MCode1/5, Write Control Instructions Generator/6(aresetn), Read Control Instructions Generator1/6(aresetn), "VDMA Interface 5.0 "/34, "VDMA Interface 5.0 "/19
  Bus Selector3/1 -> "VDMA Interface 5.0 "/20  "<awaddr>"
  Bus Selector3/2 -> "VDMA Interface 5.0 "/21  "<awalid>"
  Bus Selector3/3 -> "VDMA Interface 5.0 "/22  "<wvalid>"
  Bus Selector3/4 -> "VDMA Interface 5.0 "/23  "<wdata>"
  Bus Selector3/5 -> "VDMA Interface 5.0 "/24  "<signal5>"
  Bus Selector3/6 -> "VDMA Interface 5.0 "/25  "<signal6>"
  Bus Selector3/7 -> "VDMA Interface 5.0 "/26  "<signal7>"
  Bus Selector3/8 -> "VDMA Interface 5.0 "/27  "<signal8>"
  read_buffer_throttle/1 -> "VDMA Interface 5.0 "/28
  Bus Selector4/1 -> "VDMA Interface 5.0 "/29  "<signal1>"
  Bus Selector4/2 -> "VDMA Interface 5.0 "/30  "<signal2>"
  Bus Selector4/3 -> "VDMA Interface 5.0 "/31  "<signal3>"
  Bus Selector4/4 -> "VDMA Interface 5.0 "/32  "<signal4>"
  Bus Selector4/5 -> "VDMA Interface 5.0 "/33  "<signal5>"
  Bus Creator4/1 -> Terminator1/1
  MCode1/1 -> write_buffer_ready/1
  [s2mm_fsync_out] -> MCode1/1
  [s2mm_tready_internal] -> MCode1/2
  MCode1/2 -> [s2mm_tvalid]
  [tvalid] -> MCode1/3
  [s2mm_tlast] -> MCode1/4
  Bus Selector/3 -> [tvalid]  "<valid>"
  [s2mm_tvalid] -> "VDMA Interface 5.0 "/11
  "VDMA Interface 5.0 "/9 -> [s2mm_tready_internal]
  Constant/1 -> "VDMA Interface 5.0 "/12
  "VDMA Interface 5.0 "/32 -> Terminator2/1

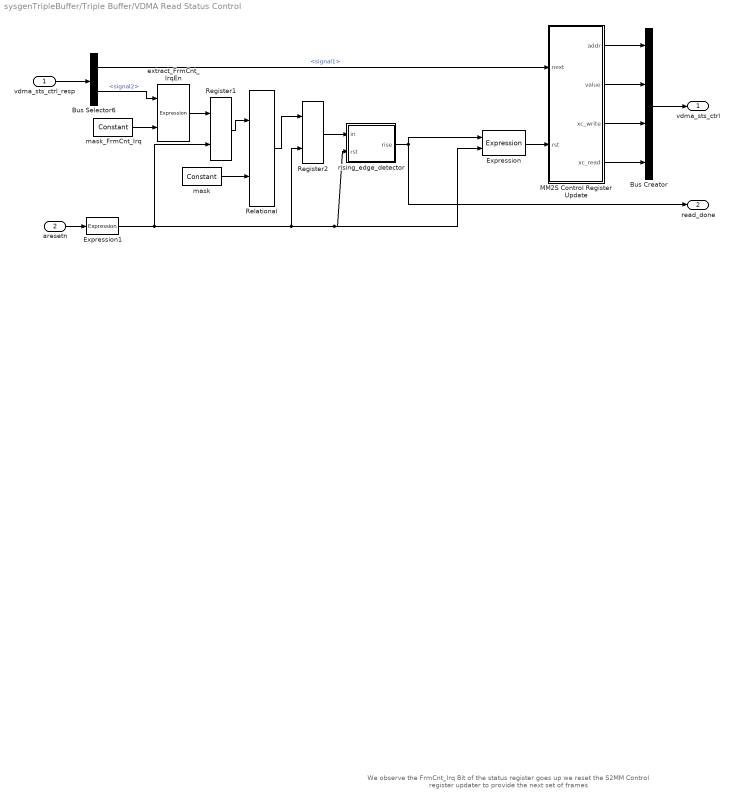
== system sysgenTripleBuffer/Triple Buffer/VDMA Read Status Control ==
  note: We observe the FrmCnt_Irq Bit of the status register goes up
      | we reset the S2MM Control register updater to provide the next
      | set of frames
  vdma_sts_ctrl_resp : Inport
  aresetn : Inport  Port=2
  Bus Creator : BusCreator
  Bus Selector6 : BusSelector  OutputSignals=signal1,signal2
  Expression : xbsIndex_r4/Expression  expression=a | b  align_bp=on  en=off  latency=0  precision=Full  arith_type=Unsigned  n_bits=16  bin_pt=0  dbl_ovrd=off  block_type=expr
      settings: block_version=12.3
  Expression1 : xbsIndex_r4/Expression  expression=~a  align_bp=on  en=off  latency=0  precision=Full  arith_type=Unsigned  n_bits=16  bin_pt=0  dbl_ovrd=off  block_type=expr
      settings: block_version=13.4
  MM2S Control Register Update : Subsystem
  Register1 : xbsIndex_r4/Register  init=0  rst=on  en=off  dbl_ovrd=off  block_type=register
      settings: block_version=12.3
  Register2 : xbsIndex_r4/Register  init=0  rst=on  en=off  dbl_ovrd=off  block_type=register
      settings: block_version=12.3
  Relational : xbsIndex_r4/Relational  mode=a=b  en=off  latency=1  dbl_ovrd=off  block_type=relational
      settings: block_version=12.3
  extract_FrmCnt_IrqEn : xbsIndex_r4/Expression  expression=a & b  align_bp=on  en=off  latency=0  precision=Full  arith_type=Unsigned  n_bits=16  bin_pt=0  dbl_ovrd=off  block_type=expr
      settings: block_version=12.3
  mask : xbsIndex_r4/Constant  const=hex2dec('00001000')  gui_display_data_type=Fixed-point  arith_type=Unsigned  n_bits=32  bin_pt=0  preci_type=Single  exp_width=8  frac_width=24  explicit_period=on  period=pixel_period  equ=P=C  opselect=C  inp2=PCIN>>17  opr=+  inp1=P  carry=CIN  dbl_ovrd=off  block_type=constant
      settings: block_version=12.3
  mask_FrmCnt_Irq : xbsIndex_r4/Constant  const=hex2dec('00001000')  gui_display_data_type=Fixed-point  arith_type=Unsigned  n_bits=32  bin_pt=0  preci_type=Single  exp_width=8  frac_width=24  explicit_period=on  period=pixel_period  equ=P=C  opselect=C  inp2=PCIN>>17  opr=+  inp1=P  carry=CIN  dbl_ovrd=off  block_type=constant
      settings: block_version=12.3
  rising_edge_detector : Subsystem
      mask Display: disp('\lceil','texmode','on')
  vdma_sts_ctrl : Outport
  read_done : Outport  Port=2
  wires:
  vdma_sts_ctrl_resp/1 -> Bus Selector6/1
  rising_edge_detector/1(rise) -> Expression/1, read_done/1
  MM2S Control Register Update/4(xc_read) -> Bus Creator/4
  MM2S Control Register Update/3(xc_write) -> Bus Creator/3
  MM2S Control Register Update/2(value) -> Bus Creator/2
  MM2S Control Register Update/1(addr) -> Bus Creator/1
  Bus Selector6/1 -> MM2S Control Register Update/1(next)  "<signal1>"
  Relational/1 -> Register2/1
  mask/1 -> Relational/2
  extract_FrmCnt_IrqEn/1 -> Register1/1
  mask_FrmCnt_Irq/1 -> extract_FrmCnt_IrqEn/2
  Bus Selector6/2 -> extract_FrmCnt_IrqEn/1  "<signal2>"
  Bus Creator/1 -> vdma_sts_ctrl/1
  Register1/1 -> Relational/1
  Register2/1 -> rising_edge_detector/1(in)
  aresetn/1 -> Expression1/1
  Expression/1 -> MM2S Control Register Update/2(rst)
  Expression1/1 -> Register1/2, Register2/2, Expression/2, rising_edge_detector/2(rst)

== system sysgenTripleBuffer/Triple Buffer/VDMA Read Transfer Command Generator ==
  axi_read_channel_in : Inport
  readFrameNumber : Inport  Port=2
  aresetn : Inport  Port=3
  Bus Creator3 : BusCreator  Inputs=5
  Bus Selector6 : BusSelector  OutputSignals=signal1,signal2,signal3,signal4,signal5,signal6,signal7,signal8
  Transmitter Block Descriptor Generator2 : xbsIndex_r4/MCode  mfname=xlScatterGatherEngineFrameTransfer  explicit_period=off  period=1  inputsTable={'boundInpExpr'=>['','','','','','','','','','','c_image_cols','c_image_rows','c_word_size'],'inputs'=>['frame','araddr','arlen','arsize','arburst','arprot','arcache','arvalid','rready','aresetn','IMAGE_COLS','IMAGE_ROWS','WORD_SIZE']}  outputsTable={'outputs'=>['arready','rvalid','rlast','rdata','rresp'],'suppressOut'=>['off','off','off','off','off']}  dbl_ovrd=off  enable_stdout=off  enable_debug=off  suppress_output=on  defparams={'IMAGE_COLS',c_image_cols,'IMAGE_ROWS',c_image_rows,'WORD_SIZE',c_word_size}  hide_port_list={}  block_type=mcode
      settings: block_version=12.3
  axi_read_channel_out : Outport
  wires:
  Bus Selector6/1 -> Transmitter Block Descriptor Generator2/2  "<signal1>"
  Bus Selector6/2 -> Transmitter Block Descriptor Generator2/3  "<signal2>"
  Bus Selector6/3 -> Transmitter Block Descriptor Generator2/4  "<signal3>"
  Bus Selector6/4 -> Transmitter Block Descriptor Generator2/5  "<signal4>"
  Bus Selector6/5 -> Transmitter Block Descriptor Generator2/6  "<signal5>"
  Bus Selector6/6 -> Transmitter Block Descriptor Generator2/7  "<signal6>"
  Bus Selector6/7 -> Transmitter Block Descriptor Generator2/8  "<signal7>"
  Bus Selector6/8 -> Transmitter Block Descriptor Generator2/9  "<signal8>"
  Bus Creator3/1 -> axi_read_channel_out/1
  axi_read_channel_in/1 -> Bus Selector6/1
  aresetn/1 -> Transmitter Block Descriptor Generator2/10
  Transmitter Block Descriptor Generator2/1 -> Bus Creator3/1
  Transmitter Block Descriptor Generator2/2 -> Bus Creator3/2
  Transmitter Block Descriptor Generator2/3 -> Bus Creator3/3
  Transmitter Block Descriptor Generator2/4 -> Bus Creator3/4
  Transmitter Block Descriptor Generator2/5 -> Bus Creator3/5
  readFrameNumber/1 -> Transmitter Block Descriptor Generator2/1

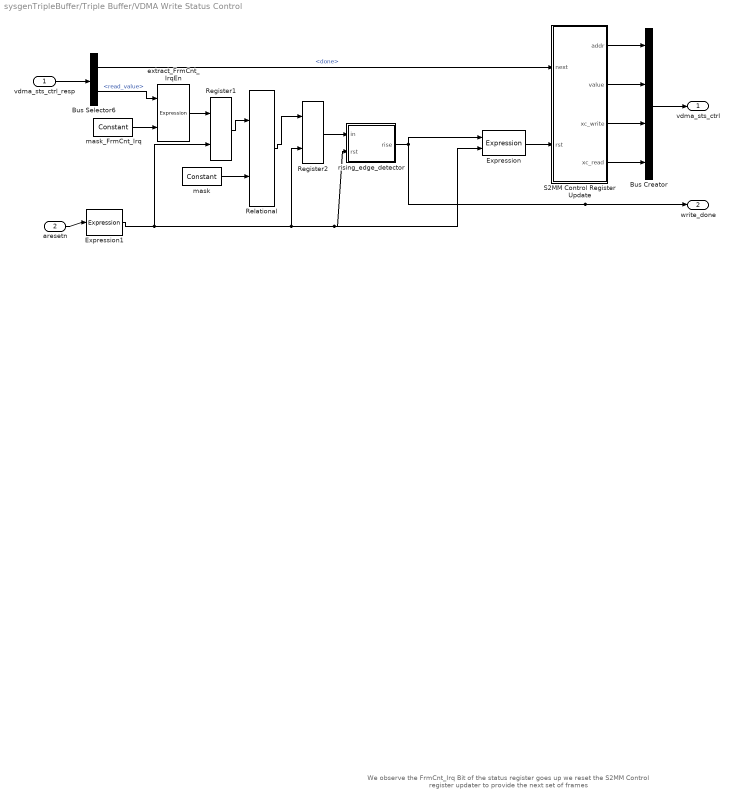
== system sysgenTripleBuffer/Triple Buffer/VDMA Write Status Control ==
  note: We observe the FrmCnt_Irq Bit of the status register goes up
      | we reset the S2MM Control register updater to provide the next
      | set of frames
  vdma_sts_ctrl_resp : Inport
  aresetn : Inport  Port=2
  Bus Creator : BusCreator
  Bus Selector6 : BusSelector  OutputSignals=done,read_value
  Expression : xbsIndex_r4/Expression  expression=a | b  align_bp=on  en=off  latency=0  precision=Full  arith_type=Unsigned  n_bits=16  bin_pt=0  dbl_ovrd=off  block_type=expr
      settings: block_version=12.3
  Expression1 : xbsIndex_r4/Expression  expression=~a  align_bp=on  en=off  latency=0  precision=Full  arith_type=Unsigned  n_bits=16  bin_pt=0  dbl_ovrd=off  block_type=expr
      settings: block_version=13.4
  Register1 : xbsIndex_r4/Register  init=0  rst=on  en=off  dbl_ovrd=off  block_type=register
      settings: block_version=12.3
  Register2 : xbsIndex_r4/Register  init=0  rst=on  en=off  dbl_ovrd=off  block_type=register
      settings: block_version=12.3
  Relational : xbsIndex_r4/Relational  mode=a=b  en=off  latency=1  dbl_ovrd=off  block_type=relational
      settings: block_version=12.3
  S2MM Control Register Update : Subsystem
  extract_FrmCnt_IrqEn : xbsIndex_r4/Expression  expression=a & b  align_bp=on  en=off  latency=0  precision=Full  arith_type=Unsigned  n_bits=16  bin_pt=0  dbl_ovrd=off  block_type=expr
      settings: block_version=12.3
  mask : xbsIndex_r4/Constant  const=hex2dec('00001000')  gui_display_data_type=Fixed-point  arith_type=Unsigned  n_bits=32  bin_pt=0  preci_type=Single  exp_width=8  frac_width=24  explicit_period=off  period=pixel_period  equ=P=C  opselect=C  inp2=PCIN>>17  opr=+  inp1=P  carry=CIN  dbl_ovrd=off  block_type=constant
      settings: block_version=12.3
  mask_FrmCnt_Irq : xbsIndex_r4/Constant  const=hex2dec('00001000')  gui_display_data_type=Fixed-point  arith_type=Unsigned  n_bits=32  bin_pt=0  preci_type=Single  exp_width=8  frac_width=24  explicit_period=off  period=pixel_period  equ=P=C  opselect=C  inp2=PCIN>>17  opr=+  inp1=P  carry=CIN  dbl_ovrd=off  block_type=constant
      settings: block_version=12.3
  rising_edge_detector : Subsystem
      mask Display: disp('\lceil','texmode','on')
  vdma_sts_ctrl : Outport
  write_done : Outport  Port=2
  wires:
  Expression1/1 -> Expression/2, rising_edge_detector/2(rst), Register2/2, Register1/2
  Expression/1 -> S2MM Control Register Update/2(rst)
  aresetn/1 -> Expression1/1
  Register2/1 -> rising_edge_detector/1(in)
  Register1/1 -> Relational/1
  Bus Creator/1 -> vdma_sts_ctrl/1
  Bus Selector6/2 -> extract_FrmCnt_IrqEn/1  "<read_value>"
  mask_FrmCnt_Irq/1 -> extract_FrmCnt_IrqEn/2
  extract_FrmCnt_IrqEn/1 -> Register1/1
  mask/1 -> Relational/2
  Relational/1 -> Register2/1
  Bus Selector6/1 -> S2MM Control Register Update/1(next)  "<done>"
  S2MM Control Register Update/1(addr) -> Bus Creator/1
  S2MM Control Register Update/2(value) -> Bus Creator/2
  S2MM Control Register Update/3(xc_write) -> Bus Creator/3
  S2MM Control Register Update/4(xc_read) -> Bus Creator/4
  rising_edge_detector/1(rise) -> Expression/1, write_done/1
  vdma_sts_ctrl_resp/1 -> Bus Selector6/1

== system sysgenTripleBuffer/Triple Buffer/VDMA Write Transfer Command Generator ==
  axi_read_channel_in : Inport
  writeFrameNumber : Inport  Port=2
  aresetn : Inport  Port=3
  Bus Creator3 : BusCreator  Inputs=5
  Bus Selector6 : BusSelector  OutputSignals=signal1,signal2,signal3,signal4,signal5,signal6,signal7,signal8
  Transmitter Block Descriptor Generator2 : xbsIndex_r4/MCode  mfname=xlScatterGatherEngineFrameTransfer  explicit_period=on  period=pixel_period  inputsTable={'boundInpExpr'=>['','','','','','','','','','','c_image_cols','c_image_rows','c_word_size'],'inputs'=>['frame','araddr','arlen','arsize','arburst','arprot','arcache','arvalid','rready','aresetn','IMAGE_COLS','IMAGE_ROWS','WORD_SIZE']}  outputsTable={'outputs'=>['arready','rvalid','rlast','rdata','rresp'],'suppressOut'=>['off','off','off','off','off']}  dbl_ovrd=off  enable_stdout=off  enable_debug=off  suppress_output=on  defparams={'IMAGE_COLS',c_image_cols,'IMAGE_ROWS',c_image_rows,'WORD_SIZE',c_word_size}  hide_port_list={}  block_type=mcode
      settings: block_version=12.3
  axi_read_channel_out : Outport
  wires:
  Bus Selector6/1 -> Transmitter Block Descriptor Generator2/2  "<signal1>"
  Bus Selector6/2 -> Transmitter Block Descriptor Generator2/3  "<signal2>"
  Bus Selector6/3 -> Transmitter Block Descriptor Generator2/4  "<signal3>"
  Bus Selector6/4 -> Transmitter Block Descriptor Generator2/5  "<signal4>"
  Bus Selector6/5 -> Transmitter Block Descriptor Generator2/6  "<signal5>"
  Bus Selector6/6 -> Transmitter Block Descriptor Generator2/7  "<signal6>"
  Bus Selector6/7 -> Transmitter Block Descriptor Generator2/8  "<signal7>"
  Bus Selector6/8 -> Transmitter Block Descriptor Generator2/9  "<signal8>"
  Bus Creator3/1 -> axi_read_channel_out/1
  aresetn/1 -> Transmitter Block Descriptor Generator2/10
  Transmitter Block Descriptor Generator2/1 -> Bus Creator3/1
  Transmitter Block Descriptor Generator2/2 -> Bus Creator3/2
  Transmitter Block Descriptor Generator2/3 -> Bus Creator3/3
  Transmitter Block Descriptor Generator2/4 -> Bus Creator3/4
  Transmitter Block Descriptor Generator2/5 -> Bus Creator3/5
  writeFrameNumber/1 -> Transmitter Block Descriptor Generator2/1
  axi_read_channel_in/1 -> Bus Selector6/1
